simulink model "CLRFSPFCRealizedSimscapeNew"  (R2024a)
settings: Solver=VariableStepAuto  StartTime=0.0  StopTime=tmax  FixedStep=tstep  MaxStep=1e-6  RelTol=1e-3  AbsTol=1e-3
undefined symbols (not defined in the file or in its folder): fg, Rc1, Rc2, Rc3, Rclp, Rin1, Rin2, Rin3, Rout, Rst1, Rst2, tmax, Vc, vr
libraries: fl_lib x46, nesl_utility x9, ee_lib x7, spsPowerLib x1, spsTHDLib x1
settings Model: Creator=FactCore  LastModifiedBy=FactCore
settings SolverCC: ZeroCrossAlgorithm=Adaptive  SolverResetMethod=Robust
settings DataIOCC: SaveTime=off
settings HardwareCC: ProdHWDeviceType=AMD->x86-64 (Windows64)
settings SFSimCC: SimTargetLang=C++

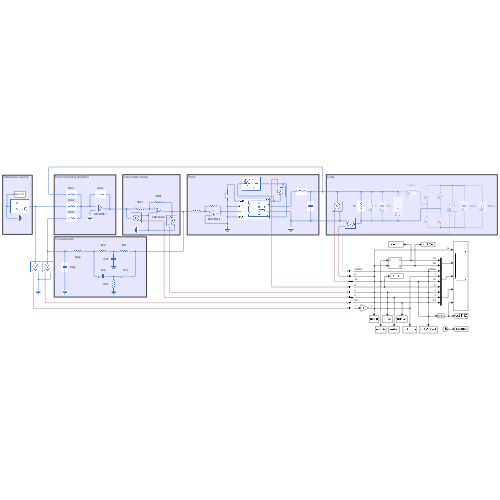
[thumbnail: Simulink's stored preview of the top-level diagram]
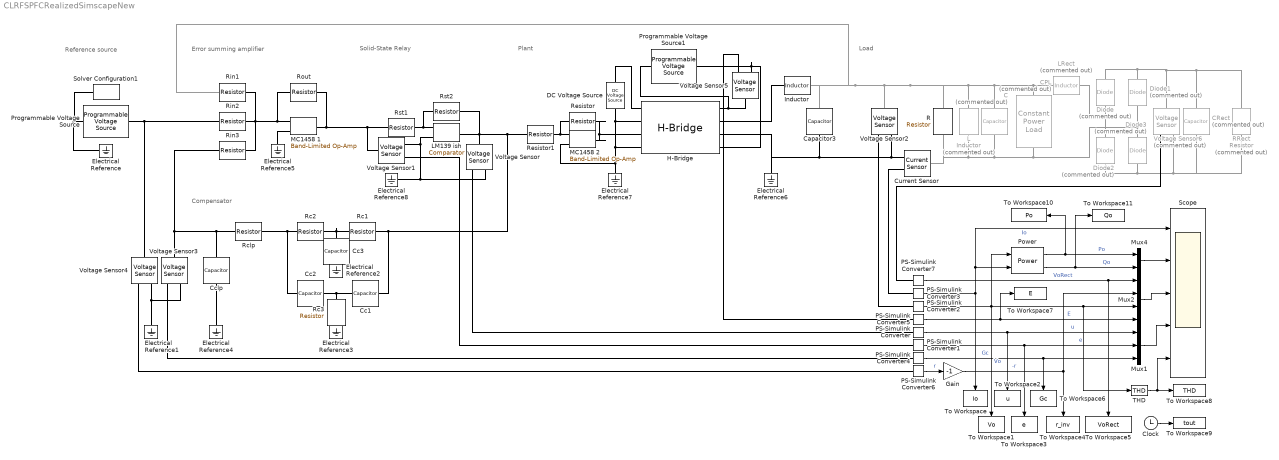
== system CLRFSPFCRealizedSimscapeNew ==
  note: Reference source
  note: Error summing amplifier
  note: Compensator
  note: Load
  note: Plant
  note: Solid-State Relay
  C : fl_lib/Electrical/Electrical Elements/Capacitor  Commented=on  c=400e-6 F  r=1e-6 Ohm  g=0 1/Ohm  i_specify=off  i_priority=None  i=0 A  i_nominal_specify=off  i_nominal_value=1  i_nominal_unit=A  v_specify=off  v_priority=None  v=0 V  v_nominal_specify=off  v_nominal_value=1  v_nominal_unit=V  vc_specify=off  vc_priority=High  vc=0 V  vc_nominal_specify=off  vc_nominal_value=1  vc_nominal_unit=V
  CPL : ee_lib/Passive/Constant Power Load  Commented=on  load_type=ee.enum.dc_ac.ac  consumed_power=100 W  min_supply_voltage=20 V  G_reverse=1e-6 S  deltaV=1e-3 V  active_power=400 W  reactive_power=0 A*V  f0=fg Hz  Vrms_min=vr*0.85 V  tau=0.01 s  Vrms_ini=vr V  Vang_ini=0 deg  enable_fault=simscape.enum.onoff.off  fault_action=simscape.enum.assert.action.none  t_fault=1 s  open_conductance=1e-4 S
      settings: InternalSimscapePortConfiguration="{\"Bottom\":[],\"Left\":[{\"id\":\"p\",\"label\":\"+\",\"type\":\"foundation.electrical.electrical\"}],\"Right\":[{\"id\":\"n\",\"label\":\"-\",\"type\":\"foundation.electrical.electrical\"}],\"Top\":[]}"
  CRect : fl_lib/Electrical/Electrical Elements/Capacitor  Commented=on  c=40e-6 F  r=1e-6 Ohm  g=0 1/Ohm  i_specify=off  i_priority=None  i=0 A  i_nominal_specify=off  i_nominal_value=1  i_nominal_unit=A  v_specify=off  v_priority=None  v=0 V  v_nominal_specify=off  v_nominal_value=1  v_nominal_unit=V  vc_specify=off  vc_priority=High  vc=0 V  vc_nominal_specify=off  vc_nominal_value=1  vc_nominal_unit=V
  Capacitor3 : fl_lib/Electrical/Electrical Elements/Capacitor  c=Cf F  r=1e-6 Ohm  g=0 1/Ohm  i_specify=off  i_priority=None  i=0 A  i_nominal_specify=off  i_nominal_value=1  i_nominal_unit=A  v_specify=off  v_priority=None  v=0 V  v_nominal_specify=off  v_nominal_value=1  v_nominal_unit=V  vc_specify=off  vc_priority=High  vc=0 V  vc_nominal_specify=off  vc_nominal_value=1  vc_nominal_unit=V
  Cc1 : fl_lib/Electrical/Electrical Elements/Capacitor  c=Cc1 F  r=1e-6 Ohm  g=0 1/Ohm  i_specify=off  i_priority=None  i=0 A  i_nominal_specify=off  i_nominal_value=1  i_nominal_unit=A  v_specify=off  v_priority=None  v=0 V  v_nominal_specify=off  v_nominal_value=1  v_nominal_unit=V  vc_specify=off  vc_priority=High  vc=0 V  vc_nominal_specify=off  vc_nominal_value=1  vc_nominal_unit=V
  Cc2 : fl_lib/Electrical/Electrical Elements/Capacitor  c=Cc2 F  r=1e-6 Ohm  g=0 1/Ohm  i_specify=off  i_priority=None  i=0 A  i_nominal_specify=off  i_nominal_value=1  i_nominal_unit=A  v_specify=off  v_priority=None  v=0 V  v_nominal_specify=off  v_nominal_value=1  v_nominal_unit=V  vc_specify=off  vc_priority=High  vc=0 V  vc_nominal_specify=off  vc_nominal_value=1  vc_nominal_unit=V
  Cc3 : fl_lib/Electrical/Electrical Elements/Capacitor  c=Cc3 F  r=1e-6 Ohm  g=0 1/Ohm  i_specify=off  i_priority=None  i=0 A  i_nominal_specify=off  i_nominal_value=1  i_nominal_unit=A  v_specify=off  v_priority=None  v=0 V  v_nominal_specify=off  v_nominal_value=1  v_nominal_unit=V  vc_specify=off  vc_priority=High  vc=0 V  vc_nominal_specify=off  vc_nominal_value=1  vc_nominal_unit=V
  Cclp : fl_lib/Electrical/Electrical Elements/Capacitor  c=Cclp F  r=1e-6 Ohm  g=0 1/Ohm  i_specify=off  i_priority=None  i=0 A  i_nominal_specify=off  i_nominal_value=1  i_nominal_unit=A  v_specify=off  v_priority=None  v=0 V  v_nominal_specify=off  v_nominal_value=1  v_nominal_unit=V  vc_specify=off  vc_priority=High  vc=0 V  vc_nominal_specify=off  vc_nominal_value=1  vc_nominal_unit=V
  Clock : Clock
  Current Sensor : fl_lib/Electrical/Electrical Sensors/Current Sensor
  DC Voltage Source : fl_lib/Electrical/Electrical Sources/DC Voltage Source  v0=5 V
  Diode{,1..3} (4 alike) : fl_lib/Electrical/Electrical Elements/Diode  Commented=on  Vf=0.6 V  Ron=0.3 Ohm  Goff=1e-8 1/Ohm  i_specify=off  i_priority=None  i=0 A  i_nominal_specify=off  i_nominal_value=1  i_nominal_unit=A  v_specify=off  v_priority=None  v=0 V  v_nominal_specify=off  v_nominal_value=1  v_nominal_unit=V
  Electrical Reference{,1..8} (9 alike) : fl_lib/Electrical/Electrical Elements/Electrical Reference
  Gain : Gain  Gain=-1
  H-Bridge : ee_lib/Semiconductors & Converters/Converters/H-Bridge  supply_ports=ee.enum.supply_ports.showsupply  pwm_or_av=ee.enum.pwm_or_av.pwm  regenerative_braking_mode=ee.enum.converters.regenerative_braking_mode.depends_on_rev  discontinuous=ee.enum.current_profile.continuous  freewheeling_mode=ee.enum.converters.freewheeling_mode.one_switch_one_diode  Rload=10 Ohm  Lload=1e-5 H  F=10 kHz  Venable=2.5 V  Vmax=5.0 V  Vreverse=0.1 V  Vbrake=2.5 V  Vm=12 V  Ron=0.1 Ohm  Don=0.05 Ohm  Goff=1e-6 S  Tmeas=298.15 K  Ron2=0.1 Ohm  Don2=0.05 Ohm  Tmeas2=398.15 K  thermal_mass=100 J/K  initial_temperature=298.15 K
      settings: InternalSimscapePortConfiguration="{\"Bottom\":[],\"Left\":[{\"id\":\"ENA\",\"label\":\"PWM\",\"type\":\"foundation.electrical.electrical\"},{\"id\":\"REF\",\"label\":\"REF\",\"type\":\"foundation.electrical.electrical\"},{\"id\":\"REV\",\"label\":\"REV\",\"type\":\"foundation.electrical.electrical\"},{\"id\":\"BRK\",\"label\":\"BRK\",\"type\":\"foundation.electrical.electrical\"}],\"Right\":[{\"id\":\"p1\",\"label\":\"V+\",\"type\":\"foundation.electrical.electrical\"},{\"id\":\"p2\",\"label\":\"+\",\"type\":\"foundation.electrical.electrical\"},{\"id\":\"n2\",\"label\":\"-\",\"type\":\"foundation.electrical.electrical\"},{\"id\":\"n1\",\"label\":\"V-\",\"type\":\"foundation.electrical.electrical\"}],\"Top\":[]}"
  Inductor : fl_lib/Electrical/Electrical Elements/Inductor  l=Lf H  r=Rf Ohm  g=1e-9 1/Ohm  i_specify=off  i_priority=None  i=0 A  i_nominal_specify=off  i_nominal_value=1  i_nominal_unit=A  v_specify=off  v_priority=None  v=0 V  v_nominal_specify=off  v_nominal_value=1  v_nominal_unit=V  i_L_specify=off  i_L_priority=High  i_L=0 A  i_L_nominal_specify=off  i_L_nominal_value=1  i_L_nominal_unit=A
  L : fl_lib/Electrical/Electrical Elements/Inductor  Commented=on  l=400e-3 H  r=1 Ohm  g=1e-9 1/Ohm  i_specify=off  i_priority=None  i=0 A  i_nominal_specify=off  i_nominal_value=1  i_nominal_unit=A  v_specify=off  v_priority=None  v=0 V  v_nominal_specify=off  v_nominal_value=1  v_nominal_unit=V  i_L_specify=off  i_L_priority=High  i_L=0 A  i_L_nominal_specify=off  i_L_nominal_value=1  i_L_nominal_unit=A
  LM139 ish : ee_lib/Integrated Circuits/Comparator  V_OS=1 mV  C_IN=0 pF  V_OL=-Vc V  V_OH=Vc V  R_OUT=50 Ohm  Delay=1.3 us
      settings: InternalSimscapePortConfiguration="{\"Bottom\":[],\"Left\":[{\"id\":\"p\",\"label\":\"+\",\"type\":\"foundation.electrical.electrical\"},{\"id\":\"n\",\"label\":\"-\",\"type\":\"foundation.electrical.electrical\"}],\"Right\":[{\"id\":\"J\",\"label\":\"\",\"type\":\"foundation.electrical.electrical\"}],\"Top\":[]}"
  LRect : fl_lib/Electrical/Electrical Elements/Inductor  Commented=on  l=22e-3 H  r=100 Ohm  g=1e-9 1/Ohm  i_specify=off  i_priority=None  i=0 A  i_nominal_specify=off  i_nominal_value=1  i_nominal_unit=A  v_specify=off  v_priority=None  v=0 V  v_nominal_specify=off  v_nominal_value=1  v_nominal_unit=V  i_L_specify=off  i_L_priority=High  i_L=0 A  i_L_nominal_specify=off  i_L_nominal_value=1  i_L_nominal_unit=A
  MC1458 1 : ee_lib/Integrated Circuits/Band-Limited Op-Amp  A=50000  Rin=0.3 MOhm  Rout=75 Ohm  Vmin=-Vc V  Vmax=Vc V  Vdotmax=200000 V/s  f=1e6 Hz  V0=0 V
  MC1458 2 : ee_lib/Integrated Circuits/Band-Limited Op-Amp  A=50000  Rin=0.3 MOhm  Rout=75 Ohm  Vmin=-Vc V  Vmax=Vc V  Vdotmax=200000 V/s  f=1e6 Hz  V0=0 V
  Mux1 : Mux  Inputs=3
  Mux2 : Mux
  Mux4 : Mux  Inputs=2
  PS-Simulink Converter{,1..7} (8 alike) : nesl_utility/PS-Simulink Converter  PhysicalDomain=network_engine_domain  SubClassName=ps_output  LeftPortType=input  RightPortType=output  PseudoPeriodic=off  Frequencies=[]  VectorFormat=inherit  Unit=inherit  AffineConversion=off
  Power : spsPowerLib/Power  Freq=fg  Vinit=[0, 0]  Iinit=[0, 0]  Ts=0
  Programmable Voltage Source : ee_lib/Sources/Programmable Voltage Source  magnitude_type=ee.enum.timechanging.constant  ac_magnitude=Vg V  magn_ramp=1 V/s  magn_step=1 V  magn_modu_magn=1 V  magn_modu_freq=1 Hz  magn_t1=1 s  magn_t2=2 s  frequency_type=ee.enum.timechanging.constant  ac_frequency=fg Hz  freq_ramp=1 Hz/s  freq_step=1 Hz  freq_modu_magn=1 Hz  freq_modu_freq=1 Hz  freq_t1=1 s  freq_t2=2 s  phase_type=ee.enum.timechanging.step  ac_shift=0 deg  phase_ramp=1 deg/s  phase_step=90 deg  phase_modu_magn=1 deg  phase_modu_freq=1 Hz  phase_t1=tmax/2 s  phase_t2=tmax s  dc_type=ee.enum.timechanging.constant  dc_voltage=0 V  dc_ramp=1 V/s  dc_step=1 V  dc_modu_magn=1 V  dc_modu_freq=1 Hz  dc_t1=1 s  dc_t2=2 s  harmonic_option=0  harmonic_orders=[5, 7, 11, 13]  harmonic_ratios=[.1, .1, .1, .1]  harmonic_shifts=[0, 0, 0, 0] deg  harmonic_t1=-inf s  harmonic_t2=inf s  noise_mode=0  PSD=0 V^2/Hz  repeatability=1  auto_seed=0  user_seed=0  sample_time=1e-3 s  i_specify=off  i_priority=None  i=0 A  i_nominal_specify=off  i_nominal_value=1  i_nominal_unit=A  v_specify=off  v_priority=None  v=0 V  v_nominal_specify=off  v_nominal_value=1  v_nominal_unit=V
      settings: InternalSimscapePortConfiguration="{\"Bottom\":[],\"Left\":[{\"id\":\"p\",\"label\":\"+\",\"type\":\"foundation.electrical.electrical\"}],\"Right\":[{\"id\":\"n\",\"label\":\"-\",\"type\":\"foundation.electrical.electrical\"}],\"Top\":[]}"
  Programmable Voltage Source1 : ee_lib/Sources/Programmable Voltage Source  magnitude_type=ee.enum.timechanging.step  ac_magnitude=0 V  magn_ramp=1 V/s  magn_step=50 V  magn_modu_magn=1 V  magn_modu_freq=1 Hz  magn_t1=tmax*3/4 s  magn_t2=tmax s  frequency_type=ee.enum.timechanging.constant  ac_frequency=fg*10 Hz  freq_ramp=1 Hz/s  freq_step=1 Hz  freq_modu_magn=1 Hz  freq_modu_freq=1 Hz  freq_t1=1 s  freq_t2=2 s  phase_type=ee.enum.timechanging.constant  ac_shift=0 deg  phase_ramp=1 deg/s  phase_step=1 deg  phase_modu_magn=1 deg  phase_modu_freq=1 Hz  phase_t1=1 s  phase_t2=2 s  dc_type=ee.enum.timechanging.constant  dc_voltage=E V  dc_ramp=1 V/s  dc_step=E/4 V  dc_modu_magn=1 V  dc_modu_freq=1 Hz  dc_t1=tmax*3/4 s  dc_t2=tmax s  harmonic_option=0  harmonic_orders=[5, 7, 11, 13]  harmonic_ratios=[.1, .1, .1, .1]  harmonic_shifts=[0, 0, 0, 0] deg  harmonic_t1=-inf s  harmonic_t2=inf s  noise_mode=0  PSD=0 V^2/Hz  repeatability=1  auto_seed=0  user_seed=0  sample_time=1e-3 s  i_specify=off  i_priority=None  i=0 A  i_nominal_specify=off  i_nominal_value=1  i_nominal_unit=A  v_specify=off  v_priority=None  v=0 V  v_nominal_specify=off  v_nominal_value=1  v_nominal_unit=V
      settings: InternalSimscapePortConfiguration="{\"Bottom\":[],\"Left\":[{\"id\":\"p\",\"label\":\"+\",\"type\":\"foundation.electrical.electrical\"}],\"Right\":[{\"id\":\"n\",\"label\":\"-\",\"type\":\"foundation.electrical.electrical\"}],\"Top\":[]}"
  R : fl_lib/Electrical/Electrical Elements/Resistor  R=150 Ohm  i_specify=off  i_priority=None  i=0 A  i_nominal_specify=off  i_nominal_value=1  i_nominal_unit=A  v_specify=off  v_priority=None  v=0 V  v_nominal_specify=off  v_nominal_value=1  v_nominal_unit=V
  RRect : fl_lib/Electrical/Electrical Elements/Resistor  Commented=on  R=150 Ohm  i_specify=off  i_priority=None  i=0 A  i_nominal_specify=off  i_nominal_value=1  i_nominal_unit=A  v_specify=off  v_priority=None  v=0 V  v_nominal_specify=off  v_nominal_value=1  v_nominal_unit=V
  Rc1 : fl_lib/Electrical/Electrical Elements/Resistor  R=Rc1 Ohm  i_specify=off  i_priority=None  i=0 A  i_nominal_specify=off  i_nominal_value=1  i_nominal_unit=A  v_specify=off  v_priority=None  v=0 V  v_nominal_specify=off  v_nominal_value=1  v_nominal_unit=V
  Rc2 : fl_lib/Electrical/Electrical Elements/Resistor  R=Rc2 Ohm  i_specify=off  i_priority=None  i=0 A  i_nominal_specify=off  i_nominal_value=1  i_nominal_unit=A  v_specify=off  v_priority=None  v=0 V  v_nominal_specify=off  v_nominal_value=1  v_nominal_unit=V
  Rc3 : fl_lib/Electrical/Electrical Elements/Resistor  R=Rc3 Ohm  i_specify=off  i_priority=None  i=0 A  i_nominal_specify=off  i_nominal_value=1  i_nominal_unit=A  v_specify=off  v_priority=None  v=0 V  v_nominal_specify=off  v_nominal_value=1  v_nominal_unit=V
  Rclp : fl_lib/Electrical/Electrical Elements/Resistor  R=Rclp Ohm  i_specify=off  i_priority=None  i=0 A  i_nominal_specify=off  i_nominal_value=1  i_nominal_unit=A  v_specify=off  v_priority=None  v=0 V  v_nominal_specify=off  v_nominal_value=1  v_nominal_unit=V
  Resistor : fl_lib/Electrical/Electrical Elements/Resistor  R=10e3 Ohm  i_specify=off  i_priority=None  i=0 A  i_nominal_specify=off  i_nominal_value=1  i_nominal_unit=A  v_specify=off  v_priority=None  v=0 V  v_nominal_specify=off  v_nominal_value=1  v_nominal_unit=V
  Resistor1 : fl_lib/Electrical/Electrical Elements/Resistor  R=10e3 Ohm  i_specify=off  i_priority=None  i=0 A  i_nominal_specify=off  i_nominal_value=1  i_nominal_unit=A  v_specify=off  v_priority=None  v=0 V  v_nominal_specify=off  v_nominal_value=1  v_nominal_unit=V
  Rin1 : fl_lib/Electrical/Electrical Elements/Resistor  R=Rin1 Ohm  i_specify=off  i_priority=None  i=0 A  i_nominal_specify=off  i_nominal_value=1  i_nominal_unit=A  v_specify=off  v_priority=None  v=0 V  v_nominal_specify=off  v_nominal_value=1  v_nominal_unit=V
  Rin2 : fl_lib/Electrical/Electrical Elements/Resistor  R=Rin2 Ohm  i_specify=off  i_priority=None  i=0 A  i_nominal_specify=off  i_nominal_value=1  i_nominal_unit=A  v_specify=off  v_priority=None  v=0 V  v_nominal_specify=off  v_nominal_value=1  v_nominal_unit=V
  Rin3 : fl_lib/Electrical/Electrical Elements/Resistor  R=Rin3 Ohm  i_specify=off  i_priority=None  i=0 A  i_nominal_specify=off  i_nominal_value=1  i_nominal_unit=A  v_specify=off  v_priority=None  v=0 V  v_nominal_specify=off  v_nominal_value=1  v_nominal_unit=V
  Rout : fl_lib/Electrical/Electrical Elements/Resistor  R=Rout Ohm  i_specify=off  i_priority=None  i=0 A  i_nominal_specify=off  i_nominal_value=1  i_nominal_unit=A  v_specify=off  v_priority=None  v=0 V  v_nominal_specify=off  v_nominal_value=1  v_nominal_unit=V
  Rst1 : fl_lib/Electrical/Electrical Elements/Resistor  R=Rst1 Ohm  i_specify=off  i_priority=None  i=0 A  i_nominal_specify=off  i_nominal_value=1  i_nominal_unit=A  v_specify=off  v_priority=None  v=0 V  v_nominal_specify=off  v_nominal_value=1  v_nominal_unit=V
  Rst2 : fl_lib/Electrical/Electrical Elements/Resistor  R=Rst2 Ohm  i_specify=off  i_priority=None  i=0 A  i_nominal_specify=off  i_nominal_value=1  i_nominal_unit=A  v_specify=off  v_priority=None  v=0 V  v_nominal_specify=off  v_nominal_value=1  v_nominal_unit=V
  Scope : Scope  NumInputPorts=5
  Solver Configuration1 : nesl_utility/Solver Configuration  PhysicalDomain=network_engine_domain  SubClassName=solver  LeftPortType=input  RightPortType=generic  Tones=[]  Harmonics=[]  SimulateNoise=off  Profile=off  UseLocalSampling=off  EnableSwitchedLinearOptims=on  FrequencyDomain=off  UseCCode=off  RelTol=0.001  AbsTol=0.001  MinStep=1e-09  ToWorkspace=off  RevertToSquareIcSolve=off  NumHomotopyIterations=100  PhasorMode=off  PhasorModeNumHarmonics=1  ConsistencySolver=NEWTON_XTOL_AFTER_FTOL  IndexReductionMethod=DerivativeReplacement  DoDC=off  ResidualTolerance=1e-09  ConsistencyTolSource=GLOBAL  ConsistencyAbsTol=0.001  ConsistencyRelTol=0.001  ConsistencyTolFactor=0.001  UseLocalSolver=off  LocalSolverChoice=NE_BACKWARD_EULER_ADVANCER  ResolveIndetEquations=on  FunctionEvalNumThread=1  LocalSolverSampleTime=0.001  DoFixedCost=off  MaxNonlinIter=3  MaxModeIter=2  ComputeImpulses=off  ImpulseIterations=2  LinearAlgebra=auto  LinearAlgebraNumThread=0  EquationFormulation=NE_TIME_EF  DelaysMemoryBudget=4096  AutomaticFiltering=on  FilteringTimeConstant=0.001  PartitionStorageMethod=AS_NEEDED  PartitionMemoryBudget=1024  PartitionMethod=ROBUST  MultibodyUseLocalSolver=off  MultibodyLocalSolverChoice=ODE1  MultibodyLocalSolverSampleTime=0.001
  THD : spsTHDLib/THD  Freq=fg  Ts=0
  To Workspace : ToWorkspace  VariableName=Io  SampleTime=-1
      settings: Decimation=outDec
  To Workspace1 : ToWorkspace  VariableName=Vo  SampleTime=-1
      settings: Decimation=outDec
  To Workspace10 : ToWorkspace  VariableName=Po  SampleTime=-1
      settings: Decimation=outDec
  To Workspace11 : ToWorkspace  VariableName=Qo  SampleTime=-1
      settings: Decimation=outDec
  To Workspace2 : ToWorkspace  VariableName=u  SampleTime=-1
      settings: Decimation=outDec
  To Workspace3 : ToWorkspace  VariableName=e  SampleTime=-1
      settings: Decimation=outDec
  To Workspace4 : ToWorkspace  VariableName=r_inv  SampleTime=-1
      settings: Decimation=outDec
  To Workspace5 : ToWorkspace  VariableName=VoRect  SampleTime=-1
      settings: Decimation=outDec
  To Workspace6 : ToWorkspace  VariableName=Gc  SampleTime=-1
      settings: Decimation=outDec
  To Workspace7 : ToWorkspace  VariableName=E  SampleTime=-1
      settings: Decimation=outDec
  To Workspace8 : ToWorkspace  VariableName=THD  SampleTime=-1
      settings: Decimation=outDec
  To Workspace9 : ToWorkspace  VariableName=tout  SampleTime=-1
      settings: Decimation=outDec
  Voltage Sensor{,1..5} (6 alike) : fl_lib/Electrical/Electrical Sensors/Voltage Sensor
  Voltage Sensor6 : fl_lib/Electrical/Electrical Sensors/Voltage Sensor  Commented=on
  wires:
  PS-Simulink Converter7/1 -> Mux2/1, To Workspace5/1  "VoRect"
  PS-Simulink Converter3/1 -> Scope/1, Power/2, To Workspace/1  "Io"
  PS-Simulink Converter2/1 -> To Workspace1/1, Mux2/3, THD/1, Power/1  "Vo"
  PS-Simulink Converter/1 -> Mux1/1, To Workspace2/1  "u"
  PS-Simulink Converter1/1 -> Mux1/2, To Workspace3/1  "e"
  Gain/1 -> Mux2/2, To Workspace4/1  "-r"
  PS-Simulink Converter6/1 -> Gain/1  "r"
  PS-Simulink Converter4/1 -> Mux1/3, To Workspace6/1  "Gc"
  Mux2/1 -> Scope/3
  Mux1/1 -> Scope/4
  Power/1 -> Mux4/1, To Workspace10/1  "Po"
  Power/2 -> Mux4/2, To Workspace11/1  "Qo"
  Mux4/1 -> Scope/2
  PS-Simulink Converter5/1 -> Mux2/4, To Workspace7/1  "E"
  THD/1 -> Scope/5, To Workspace8/1
  Clock/1 -> To Workspace9/1
  connections:
  Rst1/RConn1 -- LM139 ish/LConn1 -- Rst2/LConn1
  Voltage Sensor/RConn1 -- PS-Simulink Converter/LConn1
  PS-Simulink Converter1/LConn1 -- Voltage Sensor1/RConn1
  Solver Configuration1/RConn1 -- Electrical Reference/LConn1 -- Programmable Voltage Source/RConn1
  Electrical Reference2/LConn1 -- Cc3/RConn1
  Electrical Reference3/LConn1 -- Rc3/RConn1
  H-Bridge/RConn1 -- Programmable Voltage Source1/LConn1 -- Voltage Sensor5/LConn1
  Programmable Voltage Source1/RConn1 -- Voltage Sensor5/RConn2 -- H-Bridge/RConn4
  Rc2/LConn1 -- Cc3/LConn1 -- Rc1/RConn1
  Cc1/RConn1 -- Cc2/LConn1 -- Rc3/LConn1
  Cc2/RConn1 -- Rclp/LConn1 -- Rc2/RConn1
  Voltage Sensor3/LConn1 -- Rin3/LConn1 -- Cclp/LConn1 -- Rclp/RConn1
  Voltage Sensor4/RConn2 -- Electrical Reference1/LConn1 -- Voltage Sensor3/RConn2
  Voltage Sensor/RConn2 -- Voltage Sensor1/RConn2 -- LM139 ish/LConn2 -- Electrical Reference8/LConn1
  Rin2/RConn1 -- Rin3/RConn1 -- Rin1/RConn1 -- MC1458 1/LConn2 -- Rout/LConn1
  PS-Simulink Converter2/LConn1 -- Voltage Sensor2/RConn1
  Current Sensor/RConn1 -- PS-Simulink Converter3/LConn1
  Voltage Sensor4/RConn1 -- PS-Simulink Converter6/LConn1
  Voltage Sensor3/RConn1 -- PS-Simulink Converter4/LConn1
  Diode1/LConn1 -- Current Sensor/LConn1 -- R/RConn1 -- L/RConn1 -- C/RConn1 -- CPL/RConn1 -- Diode3/RConn1
  MC1458 1/LConn1 -- Electrical Reference5/LConn1
  Rout/RConn1 -- MC1458 1/RConn1 -- Voltage Sensor1/LConn1 -- Rst1/LConn1
  Rc1/LConn1 -- Resistor1/LConn1 -- LM139 ish/RConn1 -- Voltage Sensor/LConn1 -- Rst2/RConn1 -- Cc1/LConn1
  H-Bridge/RConn2 -- Inductor/LConn1
  Voltage Sensor4/LConn1 -- Programmable Voltage Source/LConn1 -- Rin2/LConn1
  Resistor/RConn1 -- MC1458 2/RConn1 -- H-Bridge/LConn3
  Resistor1/RConn1 -- MC1458 2/LConn2 -- Resistor/LConn1
  H-Bridge/LConn2 -- DC Voltage Source/RConn1 -- MC1458 2/LConn1 -- Electrical Reference7/LConn1 -- H-Bridge/LConn4
  Current Sensor/RConn2 -- Capacitor3/RConn1 -- H-Bridge/RConn3 -- Electrical Reference6/LConn1 -- Voltage Sensor2/RConn2
  Diode2/LConn1 -- RRect/RConn1 -- CRect/RConn1 -- Voltage Sensor6/RConn2 -- Diode3/LConn1
  C/LConn1 -- L/LConn1 -- R/LConn1 -- Voltage Sensor2/LConn1 -- Capacitor3/LConn1 -- Inductor/RConn1 -- Rin1/LConn1 -- LRect/LConn1 -- CPL/LConn1
  PS-Simulink Converter7/LConn1 -- Voltage Sensor6/RConn1
  Electrical Reference4/LConn1 -- Cclp/RConn1
  DC Voltage Source/LConn1 -- H-Bridge/LConn1
  CRect/LConn1 -- Diode/RConn1 -- Diode1/RConn1 -- Voltage Sensor6/LConn1 -- RRect/LConn1
  Diode/LConn1 -- Diode2/RConn1 -- LRect/RConn1
  Voltage Sensor5/RConn1 -- PS-Simulink Converter5/LConn1
